simulink model "Drone2_simulink"  (R2024a)
settings: Solver=ode1be  StartTime=0.0  StopTime=1000  FixedStep=0.001  MaxStep=0.001  MinStep=0.00095  RelTol=1e-3
PreLoadFcn:
  | Drone_data;
model workspace: external: MATLAB File C:\Users\admin\OneDrive - Indian Institute of Technology Jodhpur\IIT JODHPUR\Research Work\Amphibious Drone\MATLAB_CODE\2025\New_Drone\Drone_1\Drone1_simulink_DataFile.m (data not in the file)
undefined symbols (not defined in the file): Environment, Newton, Raphson, Vehicle, X, Y, Z
libraries: sm_lib x1684, nesl_utility x63, slpidlib x25, eeGeneralControl x6, matrix_library x3, rllib x2, simulink x2, fl_lib x1, sharedutil x1, SignalEditorBlockLib x1
(part 16 of 17)

== matlab function Drone2_simulink/Controller/MATLAB Function1 ==
  settings: updateMethod=DISCRETE
  data: uc output; e output; x input; rho input; g input; dt input; desired input; vd output; e_dot output; vd_dot output; eta1 output; ud_new output; ld output; Dcap_out output; TCAP_out output
function [uc, e,vd, e_dot,vd_dot,eta1,ud_new,ld,Dcap_out,TCAP_out]= adaptive_controller(x,rho,g,dt,desired)
%%%% defination
% x = states [z,p,u,w,q,lf,lr,lf_dot,lr_dot]
%  m = fixed mass
% m1 = moving mass 
% IB = Inertia tensor of 3*3
% rho = water density
% g = gravity (value in m/s^2)
% AS = syringe area
% ZS = CG location of z axis in each syringe [z1 z2 z3]
% l = length of vehicle/drone
% V = volume of drone
% rb = location of center of buoyancy from body frame [rbx rby rbz];
% RG = inital location of CG from body frame[ rgx rgy rgz];
% desired = target depth and pitch angle and velocities [z z_dot pitch
% pitch_rate]
% MATfile = file of disturnace jonswap.mat
% Parameters:    1x1 structure
%             
% 
% 
% fixed mass
% warning('on','MATLAB:singularMatrix');
% warning('on','MATLAB:nearlySingularMatrix');
% warning('on','MATLAB:illConditionedMatrix');
% dbstop if warning MATLAB:singularMatrix
% dbstop if warning MATLAB:nearlySingularMatrix
% dbstop if warning MATLAB:illConditionedMatrix


persistent isavail b Dcap Tcap %ud_prev ld_dot_prev 


if isempty(isavail)
    b = [0;0];
    Dcap = zeros(3);
    Tcap = zeros(2);
   % ud_prev = zeros(3,1);
   % ld_dot_prev = zeros(3,1);
    isavail = true;
end

k1e1= 0.05; k1e2 = 1;
parameter.K1e = diag([k1e1 k1e2]); %2x2

k2e1 = 10; k2e2 = 10; k2e3 =01;
parameter.K2eta1 = diag([k2e1 k2e2 k2e3]); %3x3

k3e1 = 5; k3e2 = 6;
parameter.K3eta2 = diag([k3e1 k3e2]);

d1 = 5; d2 =5;
parameter.Del = diag([d1 d2]); %2x2

g1 = 5; g2 = 5; g3 = 5;
parameter.Gama = diag([g1 g2 g3]);

parameter.sigma = 6;

parameter.Dtrue = diag([0.04 0.08 0.05]);
parameter.Ttrue = diag([0.002 0.002]);

parameter.opts.MaxIter = 10;
parameter.opts.lambdaLM0 = 1e-6;
parameter.opts.tol_r = 1e-6;
parameter.opts.tol_beta = 1e-6;
parameter.opts.regPI = 1e-6;
parameter.opts.beta_min = 0.001;
parameter.opts.beta_max = 0.1;






m = 7.63; % fixed mass

IB = diag([0.09331 0.1703 0.2266]);
Rsyringe = 0.02; % m
V = 8.2e-3; % m3
RG = [-0.002;0;-0.005]; % distance of cg from CO
rb = [0; 0 ; 0.008]; %m volume center
l = 0.45;
ZS = [0.0273; 0.0273; 0.0273]; % m 
lb = [1 0;0 1];
%% reuirement Checks and Pre-assign values
% P = inputParser;
% %addRequired(p,'YS',@(x) isnumeric(x) && isvector(x) && numel(x)==3)
% addRequired(P,'ZS',@(x) isnumeric(x) && iscolumn(x) && numel(x) ==3)
% addRequired(P,'rb',@(x) isnumeric(x) && iscolumn(x) && numel(x)==3)
% % addRequired(P,'IB', @(x) isnumeric(X) && ismatrix(x));
% addRequired(P,'parameters',@(x) isstruct(x));
% parse(P,ZS,rb,parameter)
% %y1 = P.Results.YS(1); y2 = p.Results.YS(2); y3 = p.Results.YS(3);
% ZS = P.Results.ZS;
% rb = P.Results.rb;
% % IB = P.Results.IB;
% parameters = P.Results.parameter;

%% control gain constants

%<------- error constant -------->
% Dtrue = parameter.Dtrue;
K1 = parameter.K1e;
K2 = parameter.K2eta1;
K3 = parameter.K3eta2;
Del = parameter.Del;
gama = parameter.Gama;
sigma = parameter.sigma;
% Ttrue = parameter.Ttrue;
% opts= parameter.opts;


Asx = pi*Rsyringe*Rsyringe*1.2;
Asz = 2*Rsyringe*l*1.2;
Asp = Asz;

%% extra
AS = pi*Rsyringe^2;
arc = [1 3 5];
jr = [3 5];
%% state Identification
% [m11,n1] = size(Dtrue);
% [m22,n22] = size(Ttrue);

Z = x(1);
r=0;y =0;
p = x(2);

u = x(3);
w = x(4);
q = x(5);
vel = [u;0;w];
omega = [0;q;0];



lf = x(6);
lr = x(7);

lf_dot = x(8);
lr_dot = x(9);


% Dcap_vec = x(8:16);
% Dcap = reshape(Dcap_vec,m11,n1);
% ud_prev = [x(17);x(18);x(19)];
% ld_prev = [x(20);x(21)];
% Tcap_vec= x(22:25);
% Tcap = reshape(Tcap_vec,m22,n22);

% b=x([28 29]);
% ld_dot_prev= [lf_dot;lr_dot];
vel1 = [u;w;q];

%% Mass Matrix and coriollis matrix
Mdead = [m*eye(3) -m*skmatrix(RG); m*skmatrix(RG) IB ];  %% dead weight mass mo
Mdead11 = m*eye(3); Mdead12 = -m*skmatrix(RG); Mdead21=-Mdead12; Mdead22 = IB;
Cdead = [zeros(3)  -skmatrix(Mdead11*vel+Mdead12*omega);-skmatrix(Mdead11*vel+Mdead12*omega) -skmatrix(Mdead21*vel+Mdead22*omega)];

[MF1, MF1_dot ,CF1] = M_Mdot_C_Matrix(rho,Rsyringe,lf,lf_dot,[(l-lf)/2; 0 ; ZS(1)],[-lf_dot/2 ;0 ;0],pi,omega,vel);
[MF2, MF2_dot ,CF2] = M_Mdot_C_Matrix(rho,Rsyringe,lf,lf_dot,[(l-lf)/2; 0 ; ZS(2)],[-lf_dot/2 ;0 ;0],pi,omega,vel);
[MR, MR_dot ,CR] = M_Mdot_C_Matrix(rho,Rsyringe,lr,lr_dot,[(l-lr)/2; 0 ; ZS(3)],[-lr_dot/2 ;0 ;0],0,omega,vel);


% MF1 = added_mass_cylinder(rho,Rsyringe,lf,[0.5*(l-lf) 0 ZS(1)],pi,1,1);
% MF2 = added_mass_cylinder(rho,Rsyringe,lf,[0.5*(l-lf) 0 ZS(2)],pi,1,1);
% MR =  added_mass_cylinder(rho,Rsyringe,lr,[0.5*(l-lr) 0 ZS(3)],pi,1,1);


M = Mdead + MF1 +MF2 +MR;
C = Cdead+ CF1 +CF2+ CR;

M_dot = MF1_dot+MF2_dot+MR_dot;


% rgx = (m*RG(1)+m1*((3*l/2)-2*lf-lr)+rho*AS*lf(l-lf)-0.5*rho*AS*lr(l-lr))/M;
% rgy = (m*RG(2)+m1*(y1+y2+y3)+2*rho*AS*lf*(y1+y2)+rho*AS*lr*y3)/M;
% rgz = (m*RG(3)+(3*m1+rho*AS*(2*lf+lr))*z1)/M;
% 
% rg = [rgx; rgy; rgz];  %% location of CG from base frame



invM =  Mdead\eye(6); %(M+0.001*eye(6))\eye(6);

M = M(arc,arc);
M_dot = M_dot(arc,arc);
invM = invM(arc,arc);
C = C(arc,arc);



%% Making Transformation matrix

Rbw = [cos(p)*cos(y) sin(r)*sin(p)*cos(y)-cos(r)*sin(y)  cos(r)*sin(p)*cos(y)+sin(r)*sin(y);
    cos(p)*sin(y) sin(r)*sin(p)*sin(y)+cos(r)*cos(y)  cos(r)*sin(p)*sin(y)-sin(r)*cos(y);
    -sin(p) sin(r)*cos(p) cos(r)*cos(p)];

Tbw = [1 sin(r)*tan(p) cos(r)*tan(p); 0 cos(r) -sin(r); 0 sin(r)/cos(p) cos(r)/cos(p)];

J = [Rbw zeros(3); zeros(3) Tbw]; % 6*6 matrix

J = J(jr,arc); %2*3 matrix [-sin(p) cos(p) 0; 0 0 1]
invJ = pinv(J); % or simply j' as J*ji  = I2;      3*2 matrix 

Jdot = [-cos(p)*q -sin(p)*q 0; 0 0 0];

%% Gravity Matrix
Fgn = [0;0;-Mdead(1,1)*g];
Fbn = [0;0;rho*V*g];

Fgb = Rbw'*Fgn;
Fbb = Rbw'*Fbn;

G = -[Fgb+Fbb; cross(RG,Fgb)+cross(rb,Fbb)]; % 6*1 matrix
G = G(arc); % 3*1 vector

%% Disturbance term
% [dx, dy, dz] = jonswapVelocitycode(t,Z,MaxOceanCurrent,MATfile);
% D= Rbw'*[dx;dy;dz];
% d= [D;0;0;0]; % 6*6 matrix
% d= d(arc);  % 3*1 vector

%% desired 
zd = desired(1);
pd = desired(2);

eta_dot_d = [desired(3);desired(4)];
eta_ddot_d = [desired(5);desired(6)];


%% error term
e= [Z;p]-[zd; pd];



%% first virtual controller \vd


vd = invJ*(eta_dot_d -K1*e);

eta1 = vel1 - vd;


e_dot = 1*J*eta1-K1*e;

vd_dot = -invJ*Jdot*invJ*(eta_dot_d-K1*e)+invJ*(eta_ddot_d-K1*e_dot);



%% second virtual controller u

fx = [0.5*Asx*rho*norm([vel1(1) vel1(2)])*x(1);0.5*Asz*rho*norm([vel(1) vel(2)])*x(2);0.5*Asp*rho*vel1(3)*vel1(3)*l];


ud_new = (C*vel1+G + Dcap*fx - 1*(pinv(eta1')*e'*J*eta1)-K2*eta1+M*vd_dot);  %% tau desired (pinv(eta1')*e'*J*eta1)

% ud_dot = (ud_new-ud_prev)/dt;

%% last controller uc
% h_fun = @(zz,ll) [(MF1(1,1)+MF2(1,1)+MR(1,1))*g*sin(zz); 
%     -(MF1(1,1)+MF2(1,1)+MR(1,1))*g*cos(zz); 
%     (MF1(1,1)+MF2(1,1))*g*(cos(zz)*((l-ll(1))/2)+ZS(1)*sin(zz))+(MR(1,1))*g*(cos(zz)*(-(l-ll(2))/2)+ZS(3)*sin(zz))];
% 
% Jh_func = @(zz,ll) [rho*g*AS*2*sin(zz) rho*g*AS*sin(zz); -rho*g*2*cos(zz) -rho*g*AS*cos(zz); rho*g*AS*((l-2*ll(1))*cos(zz)+2*ZS(1)*sin(zz))  rho*g*AS*(0.5*(l-2*ll(2))*cos(zz)+ZS(3)*sin(zz)) ];



%                   .beta_min    (optional box constraint)
%                   .beta_max
% opts.MaxIter = 10;        %    .maxIter     (default 10)
% opts.lambdaLM0 = 1e-6;    %    .lambdaLM0   (default 1e-6)
% opts.tol_r = 1e-6;        %    .tol_r       (default 1e-6)
% opts.tol_beta = 1e-6;     %    .tol_beta    (default 1e-6)
% opts.regPI = 1e-6;        %    .regPI       (default 1e-6)

%%

ld= solvebeta(AS,rho,g,l,MF1,MF2,MR,ZS,p,ud_new,[0.005; 0.005],parameter.opts);
ld = clip(ld,0.001,0.1);

% Jl = Jh_func(p,ld);

% invJl = pinv(Jl);


% Jn = [(MF1(1,1)+MF2(1,1)+MR(1,1))*g*cos(p); (MF1(1,1)+MF2(1,1)+MR(1,1))*g*sin(p);  
    % (MF1(1,1)+MF2(1,1))*g*(-sin(p)*((l-ld(1))/2)+ZS(1)*cos(p))+(MR(1,1))*g*(-sin(p)*(-(l-ld(2))/2)+ZS(3)*cos(p))];

% ld_dot = invJl*(ud_dot-Jn*q);

bb_dot = -lb*(b-ld);


l_vec = [lf;lr];
eta2 = l_vec-ld;

eta2 =reshape(eta2,2,1);
%% actual control
uc = -l_vec+Tcap*bb_dot-K3*eta2;


bbx = bb_dot*dt;
b = b+bbx;
%% State space model function
Dcap_dot = -gama*eta1*fx'-sigma.*(gama*Dcap);
Dcap_update = Dcap_dot*dt;
Dcap = Dcap+Dcap_update;
Dcap_out = Dcap;

% Defensive checks (will throw informative error)
assert(all(size(Del) == [2,2]), 'Del must be 2x2');
assert(all(size(eta2) == [2,1]), 'eta2 must be 2x1');
% disp(['size INVM = ', mat2str(size(invM))]);
% disp(['size C = ', mat2str(size(C))]);
% disp(['size vel1 = ', mat2str(size(vel1))]);
% disp(['size G = ', mat2str(size(G))]);
% disp(['size dcap = ', mat2str(size(Dcap))]);
% disp(['size fx = ', mat2str(size(fx))]);
% disp(['size pinveta1 = ', mat2str(pinv(eta1'))]);
% disp(['size edash = ', mat2str(size(e'))]);
% disp(['size J = ', mat2str(size(J))]);
% disp(['size eta1 = ', mat2str(size(eta1))]);
% disp(['size K2 = ', mat2str(size(K2))]);
% disp(['size M = ', mat2str(size(M))]);
% disp(['size vd_dot = ', mat2str(size(vd_dot))]);

assert(all(size(bb_dot) == [2,1]), 'bb_dot must be 2x1');

Tcap_dot = -Del*eta2*transpose(bb_dot);
Tcap_update = Tcap_dot*dt;
Tcap = Tcap+ Tcap_update;
TCAP_out = Tcap;




% Dcap_vect = Dcap_dot(:);
% ud_dot = ud_dot*dt;
% ld_dot = ld_dot*dt;
% tcap_vec = Tcap_dot(:);
% ld_ddot = (ld_dot-ld_dot_prev);


%% 
% ud_prev = ud_new;



end
% dx = [J*vel1; 
%     invM*(ud_new - C*vel1-G-Dtrue*fx +d);
%     Ttrue\(-l_vec+uc);
%     Dcap_dot(:);
%     ud_dot;
%     ld_dot;
%     Tcap_dot(:);
%     (ld_dot-ld_dot_prev)/dt];


function [A] = skmatrix(r)

assert(isnumeric(r),'r must be numeric');
assert(isvector(r),'r must be a vector');
assert(numel(r)==3,'length of r must be 3')


A = [0    -r(3)   r(2);
     r(3)   0    -r(1);
    -r(2)  r(1)    0];
end


function [M , M_dot, C] = M_Mdot_C_Matrix(rho, radius, length,l_dot, r_vec,r_dot, theta,omega,vlin)
% Calculate the 6x6 added mass matrix of a cylinder (general case)
%
% Inputs:
%   rho          - Fluid density
%   radius       - Cylinder radius [m]
%   length       - Cylinder length [m] 
%   l_dot        - rate of change of cylinder length
%   r_vec        - 3x1 vector from reference point (body COM) to cylinder COM [m]
%   r_dot        - 3x1 vector d(r_vec)/dt
%   Theta        - Angle of z axis roatation to make axis aline in radian (cylinder local -> body frame)
%   omega        - 3x1 vector of angular velocity  in body frame
%   vlin         - 3x1 vector of linear velocity in body frame 
% Output:
%   M      - 6x6 mass matrix in body frame 
%   M_dot  - 6x6 m_dot matrix in body frame 
%  C       - 6x6 coriolis matrix in body frame 



%% checks


assert(size(r_dot,2)==1 && size(r_dot,1)==3,'r_dot must a 3x1 numreic column vector');
assert(size(r_vec,2)==1 && size(r_vec,1)==3,'r_dot must a 3x1 numreic column vector');
assert(size(omega,2)==1 && size(omega,1)==3,'r_dot must a 3x1 numreic column vector');
assert(size(vlin,2)==1 && size(vlin,1)==3,'r_dot must a 3x1 numreic column vector');



% Volume of cylinder
V = pi * radius^2 * length;

% theta = deg2rad(theta);
R = [cos(theta) -sin(theta) 0;
    sin(theta) cos(theta) 0;
    0 0 1];

% Displaced fluid mass
m_disp = rho * V;

% Linear added mass matrix (local frame)
% Axial direction: x-axis of cylinder
% Transverse directions: y,z axes
M11_local = eye(3) * m_disp;

% Added inertia of fluid about cylinder COM in local frame
% Use standard moments of inertia formulas for a solid cylinder filled with fluid mass (added mass)
% Here, assuming fluid added mass distributed as cylinder mass with coefficients
% For fluid added inertia, multiply by coefficients as well

% Moments of inertia of solid cylinder about its center along principal axes
I_xx = 0.5 * m_disp * radius^2;                   % about cylinder axis (axial)
I_yy = (1/12) * m_disp * (3*radius^2 + length^2); % about transverse axis y
I_zz = I_yy;                                      % about transverse axis z

% Multiply moments by added mass coefficients
I_g_local = diag([I_xx, I_yy, I_zz]);

% Construct cross product matrix of r_vec
S_r = skmatrix(r_vec);

% Cross coupling matrices
M12 = m_disp * S_r;
M21 = -M12;

% Rotate inertia to body frame
I_new = R * I_g_local * R';

% Apply parallel axis theorem to inertia matrix about reference point
I_b = I_new + m_disp * (S_r * S_r');

% Rotate linear added mass matrix to body frame as well
M11 = R * M11_local * R';

% Assemble full 6x6 added mass matrix
M = [M11, M12;
     M21, I_b];



%% calculation of M dot

m1dot = rho*pi * radius^2 *l_dot;
M11dot_local = m1dot*eye(3);
M11dot = R*M11dot_local*R';
M12dot = -m1dot*skmatrix(r_vec)-m_disp*skmatrix(r_dot);
M21dot = -M12;

Ixx_dot = 0.5*rho*pi*radius^2*l_dot;
Iyy_dot = 1/12*(m1dot*(3*(r_vec'*r_vec)+length*length)+m_disp*(2*l_dot));
Izz_dot = Iyy_dot;

Idot_global = diag([Ixx_dot, Iyy_dot, Izz_dot]);


Idot = R*Idot_global*R';

M22dot = Idot + m1dot*(r_vec'*r_vec*eye(3)-r_vec*r_vec')+m_disp*(2*r_vec'*r_dot*eye(3) - (r_dot*r_vec'+r_vec*r_dot'));



M_dot = [M11dot M12dot; M21dot M22dot];


%% calcu lation of C


S_om = skmatrix(omega);
S_v = skmatrix(vlin);

adT = [S_om -S_v; zeros(3) S_om];

C = adT*M+ M_dot;


end


function beta = solvebeta(AS,rho,g,l,MF1,MF2,MR,ZS,theta, v, beta0, opts)
%SOLVE_BETA  Solve h(x, beta) = v for beta using Newton + LM + fallback
%
%   Inputs:
%       h_fun  : function handle, h_fun(x, beta) returns 2x1 vector
%       Jh_fun : function handle, Jh_fun(x, beta) returns 2x2 Jacobian wrt beta
%       x      : system state
%       v      : desired virtual input
%       beta0  : warm-start initial guess (2x1)
%       opts   : options struct with fields:
%                   .maxIter     (default 10)
%                   .tol_r       (default 1e-6)
%                   .tol_beta    (default 1e-6)
%                   .lambdaLM0   (default 1e-6)
%                   .regPI       (default 1e-6)
%                   .beta_min    (optional box constraint)
%                   .beta_max
%
%   Outputs:
%       beta   : solved beta
%       info   : struct with fields:
%                   .iterations
%                   .residual
%                   .converged
%                   .usedFallback
%
%   Jay's UAV–AUV Hybrid Control Project (PHD_DRONE)
%   ----------------------------------------------------

% h_fun = [(MF1(1,1)+MF2(1,1)+MR(1,1))*g*sin(theta);  -(MF1(1,1)+MF2(1,1)+MR(1,1))*g*cos(theta); (MF1(1,1)+MF2(1,1))*g*(cos(theta)*((l-beta_trial(1))/2)+ZS(1)*sin(theta))+(MR(1,1))*g*(cos(theta)*(-(l-beta_trial(2))/2)+ZS(3)*sin(theta))];

% Jh_func = [rho*g*AS*2*sin(theta) rho*g*AS*sin(theta); -rho*g*2*cos(theta) -rho*g*AS*cos(theta); rho*g*AS*((l-2*beta(1))*cos(zz)+2*ZS(1)*sin(theta))  rho*g*AS*(0.5*(l-2*beta(2))*cos(theta)+ZS(3)*sin(theta)) ];


%% Default options
if ~isfield(opts,'MaxIter');    opts.MaxIter  = 10;     end
if ~isfield(opts,'tol_r');      opts.tol_r    = 1e-6;   end
if ~isfield(opts,'tol_beta');   opts.tol_beta = 1e-6;   end
if ~isfield(opts,'lambdaLM0');  opts.lambdaLM0 = 1e-6;  end
if ~isfield(opts,'regPI');      opts.regPI    = 1e-6;   end

beta = beta0;
lambda = opts.lambdaLM0;
% usedFallback = false;

%% Iterative solve
for k = 1:opts.MaxIter
    
    r = [(MF1(1,1)+MF2(1,1)+MR(1,1))*g*sin(theta);  -(MF1(1,1)+MF2(1,1)+MR(1,1))*g*cos(theta); (MF1(1,1)+MF2(1,1))*g*(cos(theta)*((l-beta(1))/2)+ZS(1)*sin(theta))+(MR(1,1))*g*(cos(theta)*(-(l-beta(2))/2)+ZS(3)*sin(theta))] - v;           % residual
    if norm(r) < opts.tol_r
        break;
    end
    
    % Jacobian 2x3
    J = [rho*g*AS*2*sin(theta) rho*g*AS*sin(theta); -rho*g*2*cos(theta) -rho*g*AS*cos(theta); rho*g*AS*((l-2*beta(1))*cos(theta)+2*ZS(1)*sin(theta))  rho*g*AS*(0.5*(l-2*beta(2))*cos(theta)+ZS(3)*sin(theta)) ];
    
    % LM step: (J'J + lambda I) delta = -J' r
    % lambda = max(lambda, 1e-6);   % keeps it from becoming too small

    A = J'*J + lambda * eye(2);
    % A = A+ 1e-8*eye(2); 
    gg = J' * r;
    
   if rcond(A) < 1e-12 || any(isnan(A(:))) || any(isinf(A(:)))
       delta = -pinv(A) * gg;
   else
       delta = -A \ gg;
   end
%% SVD decomposition method
    % [U, S, V] = svd(J, 'econ');
    % S_d = diag(S);
    % S_reg = S_d ./ (S_d.^2 + lambda);   % LM update in SVD domain
    % delta = -V * diag(S_reg) * U' * r;

    
    
    % delta = -A \ g;
    beta_trial = beta + delta;
    
    % Enforce optional bounds
    if isfield(opts,'beta_min')
        beta_trial = max(beta_trial, opts.beta_min);
    end
    if isfield(opts,'beta_max')
        beta_trial = min(beta_trial, opts.beta_max);
    end
    
    % Check residual improvement
    r_trial = [(MF1(1,1)+MF2(1,1)+MR(1,1))*g*sin(theta);  -(MF1(1,1)+MF2(1,1)+MR(1,1))*g*cos(theta); (MF1(1,1)+MF2(1,1))*g*(cos(theta)*((l-beta_trial(1))/2)+ZS(1)*sin(theta))+(MR(1,1))*g*(cos(theta)*(-(l-beta_trial(2))/2)+ZS(3)*sin(theta))] - v;
    
    if norm(r_trial) < norm(r)       % accept step
        beta = beta_trial;
        lambda = lambda / 10;
        
        if norm(delta) < opts.tol_beta
            break;
        end
        
    else                             % reject step
        lambda = lambda * 10;
        
        % If lambda becomes huge → fallback
        if lambda > 1e6
            % usedFallback = true;
            % Regularized pseudo-inverse step
            delta_pi = -(J'*J + opts.regPI*eye(2)) \ (J'*r);
            beta = beta + delta_pi;
            break;
        end
    end
end

%% Prepare info
% info.iterations = k;
% info.residual = norm([(MF1(1,1)+MF2(1,1)+MR(1,1))*g*sin(theta);  -(MF1(1,1)+MF2(1,1)+MR(1,1))*g*cos(theta); (MF1(1,1)+MF2(1,1))*g*(cos(theta)*((l-beta(1))/2)+ZS(1)*sin(theta))+(MR(1,1))*g*(cos(theta)*(-(l-beta(2))/2)+ZS(3)*sin(theta))]-v);
% % info.converged = info.residual < opts.tol_r;
% info.usedFallback = usedFallback;

end

function y =clip(x,Max,Min)
y = min(Max,max(x,Min));
end

== matlab function Drone2_simulink/Controller1/Controller ==
  settings: updateMethod=DISCRETE  sampleTime=0.001
  data: state input; uc output; desired input; ld output; e output; Dcap_out output; TCAP_out output; ud_new output; bb_dot output; eta2 output; k1e1 parameter; k1e2 parameter; k2e1 parameter; k2e2 parameter; k2e3 parameter; k3e1 parameter; k3e2 parameter; d1 parameter; d2 parameter; g1 parameter; g2 parameter; g3 parameter; sigma parameter; m parameter; IB parameter; Rsyringe parameter; RG parameter; rb parameter; l parameter; ZS parameter; lb parameter; MaxIter parameter; lambdaLM0 parameter; tol_r parameter; tol_beta parameter; minb parameter; maxb parameter; Sden parameter; rho parameter; dt parameter; g parameter; MaxBuoyancyVol parameter
function [uc, ld,e,Dcap_out,TCAP_out,ud_new,bb_dot,eta2] = Adaptive_Robust_Controller(state,desired, k1e1, k1e2, k2e1, k2e2, k2e3, k3e1, k3e2, d1, d2, g1, g2, g3, sigma, m, IB, Rsyringe, RG, rb, l, ZS, lb,MaxIter, lambdaLM0, tol_r, tol_beta, minb, maxb,Sden, rho, dt, g, MaxBuoyancyVol)
%%%% defination
% x = states [z,p,u,w,q,lf,lr,lf_dot,lr_dot]
%  m = fixed mass
% m1 = moving mass 
% IB = Inertia tensor of 3*3
% rho = water density
% g = gravity (value in m/s^2)
% AS = syringe area
% ZS = CG location of z axis in each syringe [z1 z2 z3]
% l = length of vehicle/drone
% V = volume of drone
% rb = location of center of buoyancy from body frame [rbx rby rbz];
% RG = inital location of CG from body frame[ rgx rgy rgz];
% desired = target depth and pitch angle and velocities [z z_dot pitch
% pitch_rate]
% MATfile = file of disturnace jonswap.mat
% Parameters:    1x1 structure
%             
% 
% 
% fixed mass
% warning('on','MATLAB:singularMatrix');
% warning('on','MATLAB:nearlySingularMatrix');
% warning('on','MATLAB:illConditionedMatrix');
% dbstop if warning MATLAB:singularMatrix
% dbstop if warning MATLAB:nearlySingularMatrix
% dbstop if warning MATLAB:illConditionedMatrix


persistent isavail b Dcap Tcap %ud_prev ld_dot_prev 


if isempty(isavail)
    b = [0;0];
    Dcap = zeros(3);
    Tcap = zeros(2);
   % ud_prev = zeros(3,1);
   % ld_dot_prev = zeros(3,1);
    isavail = true;
end

% k1e1= 1; k1e2 = 1;
parameter.K1e = diag([k1e1 k1e2]); %2x2

% k2e1 = 10; k2e2 = 100; k2e3 =100;
parameter.K2eta1 = diag([k2e1 k2e2 k2e3]); %3x3

% k3e1 = 200; k3e2 = 200;
parameter.K3eta2 = diag([k3e1 k3e2]);

% d1 = 5; d2 =5;
parameter.Del = diag([d1 d2]); %2x2

% g1 = 5; g2 = 5; g3 = 0.5;
parameter.Gama = diag([g1 g2 g3]);

parameter.sigma = sigma;

parameter.Dtrue = diag([0.04 0.08 0.05]);
parameter.Ttrue = diag([0.002 0.002]);

parameter.opts.MaxIter = MaxIter;
parameter.opts.lambdaLM0 = lambdaLM0;
parameter.opts.tol_r = tol_r;
parameter.opts.tol_beta = 1e-6;
parameter.opts.regPI = tol_beta;
parameter.opts.beta_min = minb;
parameter.opts.beta_max = maxb;






% m = 7.61; % fixed mass

% IB = diag([0.09331 0.1703 0.2266]);
% Rsyringe = 0.02; % m
V = MaxBuoyancyVol; % m3
% RG = [-0.002;0;-0.005]; % distance of cg from CO
% rb = [0; 0 ; 0.008]; %m volume center
% l = 0.45;
% ZS = [0.0273; 0.0273; 0.0273]; % m 
% lb = 10*[1 0;0 1];
% rho = data(1);
Srho = Sden*rho;
g = abs(g);


%% reuirement Checks and Pre-assign values
% P = inputParser;
% %addRequired(p,'YS',@(x) isnumeric(x) && isvector(x) && numel(x)==3)
% addRequired(P,'ZS',@(x) isnumeric(x) && iscolumn(x) && numel(x) ==3)
% addRequired(P,'rb',@(x) isnumeric(x) && iscolumn(x) && numel(x)==3)
% % addRequired(P,'IB', @(x) isnumeric(X) && ismatrix(x));
% addRequired(P,'parameters',@(x) isstruct(x));
% parse(P,ZS,rb,parameter)
% %y1 = P.Results.YS(1); y2 = p.Results.YS(2); y3 = p.Results.YS(3);
% ZS = P.Results.ZS;
% rb = P.Results.rb;
% % IB = P.Results.IB;
% parameters = P.Results.parameter;

%% control gain constants

%<------- error constant -------->
% Dtrue = parameter.Dtrue;
K1 = parameter.K1e;
K2 = parameter.K2eta1;
K3 = parameter.K3eta2;
Del = parameter.Del;
gama = parameter.Gama;
sigma = parameter.sigma;
% Ttrue = parameter.Ttrue;
% opts= parameter.opts;


Asx = pi*Rsyringe*Rsyringe*1.2;
Asz = 2*Rsyringe*l*1.2;
Asp = Asz;

%% extra
AS = pi*Rsyringe^2;
arc = [1 3 5];
jr = [3 5];
%% state Identification
% [m11,n1] = size(Dtrue);
% [m22,n22] = size(Ttrue);

Z = state(1);
r=0;y =0;
p = state(2);

u = state(3);
w = state(4);
q = state(5);
vel = [u;0;w];
omega = [0;q;0];



lf = state(6);
lr = state(7);

lf_dot = state(8);
lr_dot = state(9);


% Dcap_vec = x(8:16);
% Dcap = reshape(Dcap_vec,m11,n1);
% ud_prev = [x(17);x(18);x(19)];
% ld_prev = [x(20);x(21)];
% Tcap_vec= x(22:25);
% Tcap = reshape(Tcap_vec,m22,n22);

% b=x([28 29]);
% ld_dot_prev= [lf_dot;lr_dot];
vel1 = [u;w;q];


%% Mass Matrix and coriollis matrix
Mdead = [m*eye(3) -m*skmatrix(RG); m*skmatrix(RG) IB ];  %% dead weight mass mo
Mdead11 = m*eye(3); Mdead12 = -m*skmatrix(RG); Mdead21=-Mdead12; Mdead22 = IB;
Cdead = [zeros(3)  -skmatrix(Mdead11*vel+Mdead12*omega);-skmatrix(Mdead11*vel+Mdead12*omega) -skmatrix(Mdead21*vel+Mdead22*omega)];

[MF1, MF1_dot ,CF1] = M_Mdot_C_Matrix(Srho,Rsyringe,lf,lf_dot,[(l-lf)/2; 0 ; ZS(1)],[-lf_dot/2 ;0 ;0],pi,omega,vel);
[MF2, MF2_dot ,CF2] = M_Mdot_C_Matrix(Srho,Rsyringe,lf,lf_dot,[(l-lf)/2; 0 ; ZS(2)],[-lf_dot/2 ;0 ;0],pi,omega,vel);
[MR, MR_dot ,CR] = M_Mdot_C_Matrix(Srho,Rsyringe,lr,lr_dot,[(l-lr)/2; 0 ; ZS(3)],[-lr_dot/2 ;0 ;0],0,omega,vel);


% MF1 = added_mass_cylinder(rho,Rsyringe,lf,[0.5*(l-lf) 0 ZS(1)],pi,1,1);
% MF2 = added_mass_cylinder(rho,Rsyringe,lf,[0.5*(l-lf) 0 ZS(2)],pi,1,1);
% MR =  added_mass_cylinder(rho,Rsyringe,lr,[0.5*(l-lr) 0 ZS(3)],pi,1,1);


M = Mdead + MF1 +MF2 +MR;
C = Cdead+ CF1 +CF2+ CR;

M_dot = MF1_dot+MF2_dot+MR_dot;


% rgx = (m*RG(1)+m1*((3*l/2)-2*lf-lr)+rho*AS*lf(l-lf)-0.5*rho*AS*lr(l-lr))/M;
% rgy = (m*RG(2)+m1*(y1+y2+y3)+2*rho*AS*lf*(y1+y2)+rho*AS*lr*y3)/M;
% rgz = (m*RG(3)+(3*m1+rho*AS*(2*lf+lr))*z1)/M;
% 
% rg = [rgx; rgy; rgz];  %% location of CG from base frame



invM =  Mdead\eye(6); %(M+0.001*eye(6))\eye(6);

M = M(arc,arc);
M_dot = M_dot(arc,arc);
invM = invM(arc,arc);
C = C(arc,arc);



%% Making Transformation matrix

Rbw = [cos(p)*cos(y) sin(r)*sin(p)*cos(y)-cos(r)*sin(y)  cos(r)*sin(p)*cos(y)+sin(r)*sin(y);
    cos(p)*sin(y) sin(r)*sin(p)*sin(y)+cos(r)*cos(y)  cos(r)*sin(p)*sin(y)-sin(r)*cos(y);
    -sin(p) sin(r)*cos(p) cos(r)*cos(p)];

Tbw = [1 sin(r)*tan(p) cos(r)*tan(p); 0 cos(r) -sin(r); 0 sin(r)/cos(p) cos(r)/cos(p)];

J = [Rbw zeros(3); zeros(3) Tbw]; % 6*6 matrix

J = J(jr,arc); %2*3 matrix [-sin(p) cos(p) 0; 0 0 1]
invJ = pinv(J); % or simply j' as J*ji  = I2;      3*2 matrix 

Jdot = [-cos(p)*q -sin(p)*q 0; 0 0 0];

%% Gravity Matrix
Fgn = [0;0;-Mdead(1,1)*g];
Fbn = [0;0;rho*V*g];

Fgb = Rbw'*Fgn;
Fbb = Rbw'*Fbn;

G = -[Fgb+Fbb; cross(RG,Fgb)+cross(rb,Fbb)]; % 6*1 matrix
G = G(arc); % 3*1 vector

%% Disturbance term
% [dx, dy, dz] = jonswapVelocitycode(t,Z,MaxOceanCurrent,MATfile);
% D= Rbw'*[dx;dy;dz];
% d= [D;0;0;0]; % 6*6 matrix
% d= d(arc);  % 3*1 vector

%% desired 
zd = desired(1);
pd = desired(2);

eta_dot_d = [desired(3);desired(4)];
eta_ddot_d = [desired(5);desired(6)];


e = [Z;p]-[zd;pd];

%% first virtual controller \vd


vd = invJ*(eta_dot_d -K1*e);

eta1 = vel1 - vd;


e_dot = 1*J*eta1-K1*e;

vd_dot = -invJ*Jdot*invJ*(eta_dot_d-K1*e)+invJ*(eta_ddot_d-K1*e_dot);



%% second virtual controller u
beta0 = [lf;lr];
fx = [0.5*Asx*rho*norm([vel1(1) vel1(2)])*vel1(1);0.5*Asz*rho*norm([vel(1) vel(2)])*vel1(2);0.5*Asp*rho*vel1(3)*vel1(3)*l];


ud_new = (C*vel1+G + Dcap*fx - J'*e-K2*eta1+M*vd_dot);  %% tau desired (pinv(eta1')*e'*J*eta1)


% ud_new(3) = clipfunc(ud_new(3),100,-100);
% if e(1) > 1
%     ld = [0.1; 0.1];
% 
% elseif e(1)<-1 || zd>-0.1 || Z>0
%     ld = [0.008; 0.008];
% 
% else
%     ld= solvebeta_pinv(AS,rho,g,l,MF1,MF2,MR,ZS,p,ud_new,beta0,parameter.opts);
%     ld = clip(ld,0.008,0.1);
% 
% end
    ld= solvebeta_pinv(AS,Srho,g,l,MF1,MF2,MR,ZS,p,ud_new,beta0,parameter.opts);
    % ld = clip(ld,0.008,0.1);

    bb_dot = -lb*(b-ld);
    l_vec = [lf;lr];
    eta2 = l_vec-ld;
    eta2 =reshape(eta2,2,1);
    %% actual control
    uc = l_vec+Tcap*bb_dot-K3*eta2;


    bbx = bb_dot*dt;
    b = b+bbx;


%% State space model function
Dcap_dot = -gama*eta1*fx'-sigma.*(gama*Dcap);
Dcap_update = Dcap_dot*dt;
Dcap = Dcap+Dcap_update;
Dcap_out = Dcap;

% Defensive checks (will throw informative error)
assert(all(size(Del) == [2,2]), 'Del must be 2x2');
assert(all(size(eta2) == [2,1]), 'eta2 must be 2x1');
% disp(['size INVM = ', mat2str(size(invM))]);
% disp(['size C = ', mat2str(size(C))]);
% disp(['size vel1 = ', mat2str(size(vel1))]);
% disp(['size G = ', mat2str(size(G))]);
% disp(['size dcap = ', mat2str(size(Dcap))]);
% disp(['size fx = ', mat2str(size(fx))]);
% disp(['size pinveta1 = ', mat2str(pinv(eta1'))]);
% disp(['size edash = ', mat2str(size(e'))]);
% disp(['size J = ', mat2str(size(J))]);
% disp(['size eta1 = ', mat2str(size(eta1))]);
% disp(['size K2 = ', mat2str(size(K2))]);
% disp(['size M = ', mat2str(size(M))]);
% disp(['size vd_dot = ', mat2str(size(vd_dot))]);

assert(all(size(bb_dot) == [2,1]), 'bb_dot must be 2x1');

Tcap_dot = -Del*eta2*transpose(bb_dot);
Tcap_update = Tcap_dot*dt;
Tcap = Tcap+ Tcap_update;
TCAP_out = Tcap;



end



function [A] = skmatrix(r)

assert(isnumeric(r),'r must be numeric');
assert(isvector(r),'r must be a vector');
assert(numel(r)==3,'length of r must be 3')


A = [0    -r(3)   r(2);
     r(3)   0    -r(1);
    -r(2)  r(1)    0];
end


function [M , M_dot, C] = M_Mdot_C_Matrix(rho, radius, length,l_dot, r_vec,r_dot, theta,omega,vlin)
% Calculate the 6x6 added mass matrix of a cylinder (general case)
%
% Inputs:
%   rho          - Fluid density
%   radius       - Cylinder radius [m]
%   length       - Cylinder length [m] 
%   l_dot        - rate of change of cylinder length
%   r_vec        - 3x1 vector from reference point (body COM) to cylinder COM [m]
%   r_dot        - 3x1 vector d(r_vec)/dt
%   Theta        - Angle of z axis roatation to make axis aline in radian (cylinder local -> body frame)
%   omega        - 3x1 vector of angular velocity  in body frame
%   vlin         - 3x1 vector of linear velocity in body frame 
% Output:
%   M      - 6x6 mass matrix in body frame 
%   M_dot  - 6x6 m_dot matrix in body frame 
%  C       - 6x6 coriolis matrix in body frame 



%% checks


assert(size(r_dot,2)==1 && size(r_dot,1)==3,'r_dot must a 3x1 numreic column vector');
assert(size(r_vec,2)==1 && size(r_vec,1)==3,'r_dot must a 3x1 numreic column vector');
assert(size(omega,2)==1 && size(omega,1)==3,'r_dot must a 3x1 numreic column vector');
assert(size(vlin,2)==1 && size(vlin,1)==3,'r_dot must a 3x1 numreic column vector');



% Volume of cylinder
V = pi * radius^2 * length;

% theta = deg2rad(theta);
R = [cos(theta) -sin(theta) 0;
    sin(theta) cos(theta) 0;
    0 0 1];

% Displaced fluid mass
m_disp = rho * V;

% Linear added mass matrix (local frame)
% Axial direction: x-axis of cylinder
% Transverse directions: y,z axes
M11_local = eye(3) * m_disp;

% Added inertia of fluid about cylinder COM in local frame
% Use standard moments of inertia formulas for a solid cylinder filled with fluid mass (added mass)
% Here, assuming fluid added mass distributed as cylinder mass with coefficients
% For fluid added inertia, multiply by coefficients as well

% Moments of inertia of solid cylinder about its center along principal axes
I_xx = 0.5 * m_disp * radius^2;                   % about cylinder axis (axial)
I_yy = (1/12) * m_disp * (3*radius^2 + length^2); % about transverse axis y
I_zz = I_yy;                                      % about transverse axis z

% Multiply moments by added mass coefficients
I_g_local = diag([I_xx, I_yy, I_zz]);

% Construct cross product matrix of r_vec
S_r = skmatrix(r_vec);

% Cross coupling matrices
M12 = m_disp * S_r;
M21 = -M12;

% Rotate inertia to body frame
I_new = R * I_g_local * R';

% Apply parallel axis theorem to inertia matrix about reference point
I_b = I_new + m_disp * (S_r * S_r');

% Rotate linear added mass matrix to body frame as well
M11 = R * M11_local * R';

% Assemble full 6x6 added mass matrix
M = [M11, M12;
     M21, I_b];



%% calculation of M dot

m1dot = rho*pi * radius^2 *l_dot;
M11dot_local = m1dot*eye(3);
M11dot = R*M11dot_local*R';
M12dot = -m1dot*skmatrix(r_vec)-m_disp*skmatrix(r_dot);
M21dot = -M12;

Ixx_dot = 0.5*rho*pi*radius^2*l_dot;
Iyy_dot = 1/12*(m1dot*(3*(r_vec'*r_vec)+length*length)+m_disp*(2*l_dot));
Izz_dot = Iyy_dot;

Idot_global = diag([Ixx_dot, Iyy_dot, Izz_dot]);


Idot = R*Idot_global*R';

M22dot = Idot + m1dot*(r_vec'*r_vec*eye(3)-r_vec*r_vec')+m_disp*(2*r_vec'*r_dot*eye(3) - (r_dot*r_vec'+r_vec*r_dot'));



M_dot = [M11dot M12dot; M21dot M22dot];


%% calcu lation of C


S_om = skmatrix(omega);
S_v = skmatrix(vlin);

adT = [S_om -S_v; zeros(3) S_om];

C = adT*M+ M_dot;


end


function beta = solvebeta(AS,rho,g,l,MF1,MF2,MR,ZS,theta, v, beta0, opts)
%SOLVE_BETA  Solve h(x, beta) = v for beta using Newton + LM + fallback
%
%   Inputs:
%       h_fun  : function handle, h_fun(x, beta) returns 2x1 vector
%       Jh_fun : function handle, Jh_fun(x, beta) returns 2x2 Jacobian wrt beta
%       x      : system state
%       v      : desired virtual input
%       beta0  : warm-start initial guess (2x1)
%       opts   : options struct with fields:
%                   .maxIter     (default 10)
%                   .tol_r       (default 1e-6)
%                   .tol_beta    (default 1e-6)
%                   .lambdaLM0   (default 1e-6)
%                   .regPI       (default 1e-6)
%                   .beta_min    (optional box constraint)
%                   .beta_max
%
%   Outputs:
%       beta   : solved beta
%       info   : struct with fields:
%                   .iterations
%                   .residual
%                   .converged
%                   .usedFallback
%
%   Jay's UAV–AUV Hybrid Control Project (PHD_DRONE)
%   ----------------------------------------------------

% h_fun = [(MF1(1,1)+MF2(1,1)+MR(1,1))*g*sin(theta);  -(MF1(1,1)+MF2(1,1)+MR(1,1))*g*cos(theta); (MF1(1,1)+MF2(1,1))*g*(cos(theta)*((l-beta_trial(1))/2)+ZS(1)*sin(theta))+(MR(1,1))*g*(cos(theta)*(-(l-beta_trial(2))/2)+ZS(3)*sin(theta))];

% Jh_func = [rho*g*AS*2*sin(theta) rho*g*AS*sin(theta); -rho*g*2*cos(theta) -rho*g*AS*cos(theta); rho*g*AS*((l-2*beta(1))*cos(zz)+2*ZS(1)*sin(theta))  rho*g*AS*(0.5*(l-2*beta(2))*cos(theta)+ZS(3)*sin(theta)) ];


%% Default options
if ~isfield(opts,'MaxIter');    opts.MaxIter  = 10;     end
if ~isfield(opts,'tol_r');      opts.tol_r    = 1e-6;   end
if ~isfield(opts,'tol_beta');   opts.tol_beta = 1e-6;   end
if ~isfield(opts,'lambdaLM0');  opts.lambdaLM0 = 1e-6;  end
if ~isfield(opts,'regPI');      opts.regPI    = 1e-6;   end

beta = beta0;
lambda = opts.lambdaLM0;
% usedFallback = false;

%% Iterative solve
for k = 1:opts.MaxIter
    
    r = [(MF1(1,1)+MF2(1,1)+MR(1,1))*g*sin(theta);  -(MF1(1,1)+MF2(1,1)+MR(1,1))*g*cos(theta); (MF1(1,1)+MF2(1,1))*g*(cos(theta)*((l-beta(1))/2)+ZS(1)*sin(theta))+(MR(1,1))*g*(cos(theta)*(-(l-beta(2))/2)+ZS(3)*sin(theta))] - v;           % residual
    if norm(r) < opts.tol_r
        break;
    end
    
    % Jacobian 2x3
    J = [rho*g*AS*2*sin(theta) rho*g*AS*sin(theta); -rho*g*2*AS*cos(theta) -rho*g*AS*cos(theta); rho*g*AS*((l-2*beta(1))*cos(theta)+2*ZS(1)*sin(theta))  rho*g*AS*(-0.5*(l-2*beta(2))*cos(theta)+ZS(3)*sin(theta)) ];
    
    % LM step: (J'J + lambda I) delta = -J' r
    % lambda = max(lambda, 1e-6);   % keeps it from becoming too small

    A = J'*J + lambda * eye(2);
    % A = A+ 1e-8*eye(2); 
    gg = J' * r;
    
   if rcond(A) < 1e-12 || any(isnan(A(:))) || any(isinf(A(:)))
       delta = pinv(A) * gg;
   else
       delta = A \ gg;
   end
%% SVD decomposition method
    % [U, S, V] = svd(J, 'econ');
    % S_d = diag(S);
    % S_reg = S_d ./ (S_d.^2 + lambda);   % LM update in SVD domain
    % delta = -V * diag(S_reg) * U' * r;

    
    
    % delta = -A \ g;
    beta_trial = beta + delta;
    
    % Enforce optional bounds
    if isfield(opts,'beta_min')
        beta_trial = max(beta_trial, opts.beta_min);
    end
    if isfield(opts,'beta_max')
        beta_trial = min(beta_trial, opts.beta_max);
    end
    
    % Check residual improvement
    r_trial = [(MF1(1,1)+MF2(1,1)+MR(1,1))*g*sin(theta);  -(MF1(1,1)+MF2(1,1)+MR(1,1))*g*cos(theta); (MF1(1,1)+MF2(1,1))*g*(cos(theta)*((l-beta_trial(1))/2)+ZS(1)*sin(theta))+(MR(1,1))*g*(cos(theta)*(-(l-beta_trial(2))/2)+ZS(3)*sin(theta))] - v;
    
    if norm(r_trial) < norm(r)       % accept step
        beta = beta_trial;
        lambda = lambda / 10;
        
        if norm(delta) < opts.tol_beta
            break;
        end
        
    else                             % reject step
        lambda = lambda * 10;
        
        % If lambda becomes huge → fallback
        if lambda > 1e6
            % usedFallback = true;
            % Regularized pseudo-inverse step
            delta_pi = -(J'*J + opts.regPI*eye(2)) \ (J'*r);
            beta = beta + delta_pi;
            break;
        end
    end
end
end

function beta = solvebeta_pinv(AS,rho,g,l,MF1,MF2,MR,ZS,theta, v,beta0, opts)
%SOLVE_BETA  Solve h(x, beta) = v for beta using Newton + LM + fallback
%
%   Inputs:
%       h_fun  : function handle, h_fun(x, beta) returns 2x1 vector
%       Jh_fun : function handle, Jh_fun(x, beta) returns 2x2 Jacobian wrt beta
%       x      : system state
%       v      : desired virtual input
%       beta0  : warm-start initial guess (2x1)
%       opts   : options struct with fields:
%                   .maxIter     (default 10)
%                   .tol_r       (default 1e-6)
%                   .tol_beta    (default 1e-6)
%                   .lambdaLM0   (default 1e-6)
%                   .regPI       (default 1e-6)
%                   .beta_min    (optional box constraint)
%                   .beta_max
%
%   Outputs:
%       beta   : solved beta
%       info   : struct with fields:
%                   .iterations
%                   .residual
%                   .converged
%                   .usedFallback
%
%   Jay's UAV–AUV Hybrid Control Project (PHD_DRONE)
%   ----------------------------------------------------

% h_fun = [(MF1(1,1)+MF2(1,1)+MR(1,1))*g*sin(theta);  -(MF1(1,1)+MF2(1,1)+MR(1,1))*g*cos(theta); (MF1(1,1)+MF2(1,1))*g*(cos(theta)*((l-beta_trial(1))/2)+ZS(1)*sin(theta))+(MR(1,1))*g*(cos(theta)*(-(l-beta_trial(2))/2)+ZS(3)*sin(theta))];

% Jh_func = [rho*g*AS*2*sin(theta) rho*g*AS*sin(theta); -rho*g*2*cos(theta) -rho*g*AS*cos(theta); rho*g*AS*((l-2*beta(1))*cos(zz)+2*ZS(1)*sin(theta))  rho*g*AS*(0.5*(l-2*beta(2))*cos(theta)+ZS(3)*sin(theta)) ];


%% Default options
% if ~isfield(opts,'MaxIter');    opts.MaxIter  = 10;     end
% if ~isfield(opts,'tol_r');      opts.tol_r    = 1e-6;   end
% if ~isfield(opts,'tol_beta');   opts.tol_beta = 1e-6;   end
% if ~isfield(opts,'lambdaLM0');  opts.lambdaLM0 = 1e-6;  end
% if ~isfield(opts,'regPI');      opts.regPI    = 1e-6;   end

beta = beta0;

%% Iterative solve
for k = 1:opts.MaxIter
    beta_prev = beta;
    r = [(MF1(1,1)+MF2(1,1)+MR(1,1))*g*sin(theta);  -(MF1(1,1)+MF2(1,1)+MR(1,1))*g*cos(theta); (MF1(1,1)+MF2(1,1))*g*(cos(theta)*((l-beta(1))/2)+ZS(1)*sin(theta))+(MR(1,1))*g*(cos(theta)*(-(l-beta(2))/2)+ZS(3)*sin(theta))] - v;           % residual
    
    % Jacobian 2x3
    J = [rho*g*AS*2*sin(theta) rho*g*AS*sin(theta); -rho*g*2*AS*cos(theta) -rho*g*AS*cos(theta); rho*g*AS*((l-2*beta(1))*cos(theta)+2*ZS(1)*sin(theta))  rho*g*AS*(-0.5*(l-2*beta(2))*cos(theta)+ZS(3)*sin(theta)) ];
    
    beta = beta-(J.'*J)\(J.'*r);

    r = [(MF1(1,1)+MF2(1,1)+MR(1,1))*g*sin(theta);  -(MF1(1,1)+MF2(1,1)+MR(1,1))*g*cos(theta); (MF1(1,1)+MF2(1,1))*g*(cos(theta)*((l-beta(1))/2)+ZS(1)*sin(theta))+(MR(1,1))*g*(cos(theta)*(-(l-beta(2))/2)+ZS(3)*sin(theta))] - v;           % residual

    if all(abs(beta-beta_prev) < 1e-3) && norm(r)<opts.tol_r
        break
    end


end
    
    
    % Enforce optional bounds
    if isfield(opts,'beta_min')
        for i=1:length(beta)
            beta(i) = max(beta(i), opts.beta_min);
        end
    end
    if isfield(opts,'beta_max')
        for i=1:length(beta)
            beta(i) = min(beta(i), opts.beta_max);
        end
    end 
end


%% Prepare info
% info.iterations = k;
% info.residual = norm([(MF1(1,1)+MF2(1,1)+MR(1,1))*g*sin(theta);  -(MF1(1,1)+MF2(1,1)+MR(1,1))*g*cos(theta); (MF1(1,1)+MF2(1,1))*g*(cos(theta)*((l-beta(1))/2)+ZS(1)*sin(theta))+(MR(1,1))*g*(cos(theta)*(-(l-beta(2))/2)+ZS(3)*sin(theta))]-v);
% % info.converged = info.residual < opts.tol_r;
% info.usedFallback = usedFallback;



function y =clipfunc(x,Max,Min)
y = min(Max,max(x,Min));
end

== matlab function Drone2_simulink/Hydrostatic & Hydrodynamic Effects/Drag Sub system/Hydrodyanamic drag/MATLAB Function ==
  data: u input; y output; MIN parameter; MAX parameter
function y = fcn(u,MIN, MAX)
y =zeros(length(u),1);
for i =1:length(u)
    y(i) = max(MIN,min(u(i),MAX));
end
end

== matlab function Drone2_simulink/Hydrostatic & Hydrodynamic Effects/Drag Sub system/Hydrodyanamic drag/MATLAB Function1 ==
  data: u input; y output; A parameter; B parameter
function y = fcn(u,A, B)
y =zeros(length(u),1);
for i =1:length(u)
    y(i) = max(A,min(u(i),B));
end
end

== matlab function Drone2_simulink/Controller1/RL System/MATLAB Function2 ==
  data: Obsevation input; reward output; Desired input; feedback input; Const parameter
%% reward Function
function reward = rewardFunction(Obsevation,Desired,feedback, Const)
% Target depth and pitch
depth = Observation(1);
depthRate = Obsevation(2);
pitch= Obsevation(3);
pitchRate = Obsevation(4);
Fs1pos = Obsevation(5);
Fs2pos = Obsevation(6);
Fs1vel = Obsevation(7);
Fs2vel = Obsevation(8);
Bspos = Obsevation(9);
Bsvel = Obsevation(10);
A = const;
depth_ref = Desired(1);
pitch_ref = Desired(2);



depth_error = depth - depth_ref;
pitch_error = pitch - pitch_ref;


reward = - (5 * depth_error^2 + 2 * pitch_error^2 + 0.5 * depthRate^2 + 0.5 * pitchRate^2);
end

== matlab function Drone2_simulink/Controller1/RL System/MATLAB Function3 ==
  data: Observation input; reward output; Desired input; MaxVel parameter; MaxPose parameter; MinPose parameter; Delta parameter; K parameter
%% reward Function
function reward = rewardFunction(Observation,Desired, MaxVel, MaxPose, MinPose, Delta, K)
% Target depth and pitch
depth = Observation(1);
depthRate = Observation(2);
pitch= Observation(3);
pitchRate = Observation(4);
Fs1pos = Observation(5);
Fs2pos = Observation(6);
Fs1vel = Observation(7);
Fs2vel = Observation(8);
Bspos = Observation(9);
Bsvel = Observation(10);


Syring1Reward = syringeRewardSigmoid(Fs1pos,Fs1vel,MinPose,MaxPose,Delta,MaxVel,K);
Syring2Reward = syringeRewardSigmoid(Fs2pos,Fs2vel,MinPose,MaxPose,Delta,MaxVel,K);
Syring3Reward = syringeRewardSigmoid(Bspos,Bsvel,MinPose,MaxPose,Delta,MaxVel,K);


depth_ref = Desired(1);
pitch_ref = Desired(2);



depth_error = depth - depth_ref;
pitch_error = pitch - pitch_ref;


reward = - (5 * depth_error^2 + 0.1 * pitch_error^2 + 0.25 * depthRate^2 + 0.5 * pitchRate^2+0.25*depth_error*depthRate+0.25*pitchRate*pitch_error+depth_error*((Fs1vel+Fs2vel)/2+Bsvel)) + 02*(Syring1Reward+Syring2Reward+Syring3Reward);
end


function reward = syringeRewardSigmoid(pos, vel, minPos, maxPos, delta, vmax, k)
    % Position penalty
    p1 = 1 / (1 + exp(-k * (pos - (maxPos - delta))));
    p2 = 1 / (1 + exp(k  * (pos - (minPos + delta))));
    penalty_pos = p1 + p2;

    % Velocity penalty
    penalty_vel = 1 / (1 + exp(-k * (abs(vel) - vmax)));

    % Total penalty
    total_penalty = penalty_pos + 1.2*penalty_vel;

    % Reward is negative penalty
    reward = -total_penalty;
end

== matlab function Drone2_simulink/Controller1/RL System/MATLAB Function4 ==
  data: obs input; reward output; desired input; MaxVel parameter; MaxPose parameter; MinPose parameter; Delta parameter
%% reward Function
%function reward = rewardFunction(Observation,Desired, MaxVel, MaxPose, MinPose, Delta, K)


function reward = smoothReward(obs, desired,MaxVel, MaxPose, MinPose, Delta)

    % Unpack observations
    z           = obs(1);    % depth
    z_dot       = obs(2);    % vertical speed
    pitch       = obs(3);    % pitch
    pitch_dot   = obs(4);    % pitch rate
    syrPosFL     = obs(5);    % front syringe position
    syrVelFL     = obs(6);    % front syringe velocity
    syrPosFR     = obs(7);    % back syringe position
    syrVelFR     = obs(8);    % back syringe velocity
    syrPosB     = obs(9);    % back syringe position
    syrVelB    = obs(10);    % back syringe velocity
    syrPosF = (syrPosFR+syrPosFL)/2;
    syrVelF= (syrVelFL+syrVelFR)/2;

    % Desired states
    z_des       = desired(1);
    pitch_des   = desired(2);

    % Errors
    err_z       = z-z_des;
    err_pitch   = pitch - pitch_des;

    % --- Smooth reward components ---

    % 1. Penalize total absolute error
    reward_err = - 0.5*(abs(err_z) + 0.025 * abs(err_pitch));

    % 2. Encourage corrective motion (dot product of error and velocity)
    reward_z_dot      = -0.05 * tanh(err_z * z_dot);
    reward_pitch_dot  = -0.005 * tanh(err_pitch * pitch_dot);

    % 3. Encourage syringe motion that helps depth correction
    reward_syringe_dir =  0.01*tanh(err_z * (syrVelF + syrVelB));

    % 4. Penalize being near limits of syringe stroke (soft cushion)
    minPos = MinPose; maxPos = MaxPose; cushion = Delta;

    penalty_cushionF = -0.05 * exp( - ((syrPosF - (minPos + cushion)) * (maxPos - cushion - syrPosF)) * 1e2 );
    penalty_cushionB = -0.05 * exp( - ((syrPosB - (minPos + cushion)) * (maxPos - cushion - syrPosB)) * 1e2 );

    % 5. Penalize excessive syringe velocity (soft)
    maxVel = MaxVel;
    penalty_velF = -0.1 * max(0, abs(syrVelF) - maxVel);
    penalty_velB = -0.1 * max(0, abs(syrVelB) - maxVel);

    % Final reward
    reward = reward_err + reward_z_dot + reward_pitch_dot + ...
             reward_syringe_dir + ...
             penalty_cushionF + penalty_cushionB + ...
             penalty_velF + penalty_velB;

end



% function reward = syringeRewardSigmoid(pos, vel, minPos, maxPos, delta, vmax, k)
%     % Position penalty
%     p1 = 1 / (1 + exp(-k * (pos - (maxPos - delta))));
%     p2 = 1 / (1 + exp(k  * (pos - (minPos + delta))));
%     penalty_pos = p1 + p2;
% 
%     % Velocity penalty
%     penalty_vel = 1 / (1 + exp(-k * (abs(vel) - vmax)));
% 
%     % Total penalty
%     total_penalty = penalty_pos + 1.2*penalty_vel;
% 
%     % Reward is negative penalty
%     reward = -total_penalty;
% end

== matlab function Drone2_simulink/Controller1/Underwater_Syringe_Actuation/MATLAB Function1 ==
  settings: updateMethod=DISCRETE
  data: F_b input; Z input; Zdesired input; ez input; ez_dot input; dt parameter; rho parameter; A parameter; Vf_cmd output; Vb_cmd output; Vf_trim_hat output; Vb_trim_hat output; g parameter; V_MAX parameter; V_MIN parameter; V_DOT_MAX parameter; Kp_pos parameter; Kp_vel parameter; Ez_high parameter; Kr parameter; sigma parameter
function [Vf_cmd, Vb_cmd, Vf_trim_hat, Vb_trim_hat] = ...
    syringe_allocation_adaptive_3(F_b, Z,Zdesired,ez, ez_dot, dt,rho,A,g, V_MAX, V_MIN, V_DOT_MAX, Kp_pos, Kp_vel, Ez_high, Kr, sigma)
%#codegen
% Adaptive allocation for 2-front + 1-rear syringes
% Implements depth-priority control with sigma-region energy saving
% Author: Shrivi Jay Khatri

%% --- Physical Parameters ---
% rho = 1000;     % kg/m^3
% g   = 9.81;     % m/s^2
% A   = 0.026;    % m^2 (syringe cross-section area)
% V_MIN = 0.005;  % m
% V_MAX = 0.100;  % m
% V_DOT_MAX = 0.012; % m/s (12 mm/s)
% 
% %% --- Adaptive Tuning Parameters ---
% Kp_pos = 0.25;     % proportional position gain
% Kp_vel = 0.02;     % velocity-region damping gain
% Kr     = 2.0;      % rate sensitivity (adaptive damping)
% sigma  = 0.01;     % deadband threshold (m)
% Ez_high = 0.05;    % large-error boundary (m)

%% --- Persistent Adaptive Trims ---
persistent Vf_trim Vb_trim inited
if isempty(inited)
    Vf_trim = 0.046;   % Initial trim (front, m)
    Vb_trim = 0.031;   % Initial trim (rear, m)
    inited = true;
end
if Zdesired>=0.1 || Z>0
    Vf_cmd= V_MIN;
    Vf_trim_hat = V_MIN;
    Vb_cmd = V_MIN;
    Vb_trim_hat =V_MIN;
    return
end
%% --- Compute Effective Stroke Change from Force Demand ---
dSum = F_b / (rho * g * A);   % Total stroke equivalent (2Vf + Vb)
Vf_inc = 0.25 * dSum;         % each front syringe increment
Vb_inc = 0.50 * dSum;         % rear syringe increment

%% --- Adaptive Trim Update Logic ---
if abs(ez) > Ez_high
    % Region 1: Large error → aggressive move
    dVf_trim = sign(ez) * V_DOT_MAX * dt * 0.8;
    dVb_trim = sign(ez) * V_DOT_MAX * dt * 0.8;

elseif abs(ez) > sigma
    % Region 2: Moderate error → position-based slow adaptation
    adapt_factor = 1 / (1 + Kr * abs(ez_dot));
    dSum_trim = Kp_pos * ez * adapt_factor * dt;
    dVf_trim = 0.25 * dSum_trim;
    dVb_trim = 0.50 * dSum_trim;

else
    % Region 3: Small error → velocity-based energy saving
    adapt_factor = 1 / (1 + Kr * abs(ez_dot));
    dSum_trim = -Kp_vel * ez_dot * adapt_factor * dt;
    dVf_trim = 0.25 * dSum_trim;
    dVb_trim = 0.50 * dSum_trim;
end

%% --- Update and Clamp Trims ---
Vf_trim = clamp(Vf_trim + dVf_trim, V_MIN, V_MAX);
Vb_trim = clamp(Vb_trim + dVb_trim, V_MIN, V_MAX);

%% --- Combine Trim and Fast Correction ---
Vf_target = Vf_trim + Vf_inc;
Vb_target = Vb_trim + Vb_inc;

%% --- Clamp Syringe Limits ---
Vf_cmd = clamp(Vf_target, V_MIN, V_MAX);
Vb_cmd = clamp(Vb_target, V_MIN, V_MAX);

%% --- Outputs for Observation ---
Vf_trim_hat = Vf_trim;
Vb_trim_hat = Vb_trim;

end

%% === Helper Functions ===
function y = clamp(x, xmin, xmax)
    y = min(max(x, xmin), xmax);
end
